simulink model "in_search_for_controller"  (R2017b)
settings: Solver=FixedStepDiscrete  StartTime=0.0  StopTime=10  FixedStep=0.01  RelTol=1e-3
undefined symbols (not defined in the file): g, h, lf, lr, m, r, wf, wr
libraries: vrlib x4, simulink x3, sharedtransform x1
settings Model: Creator=ashwin.ramanujam  LastModifiedBy=Lenovo g505s
settings DataIOCC: ReturnWorkspaceOutputs=on

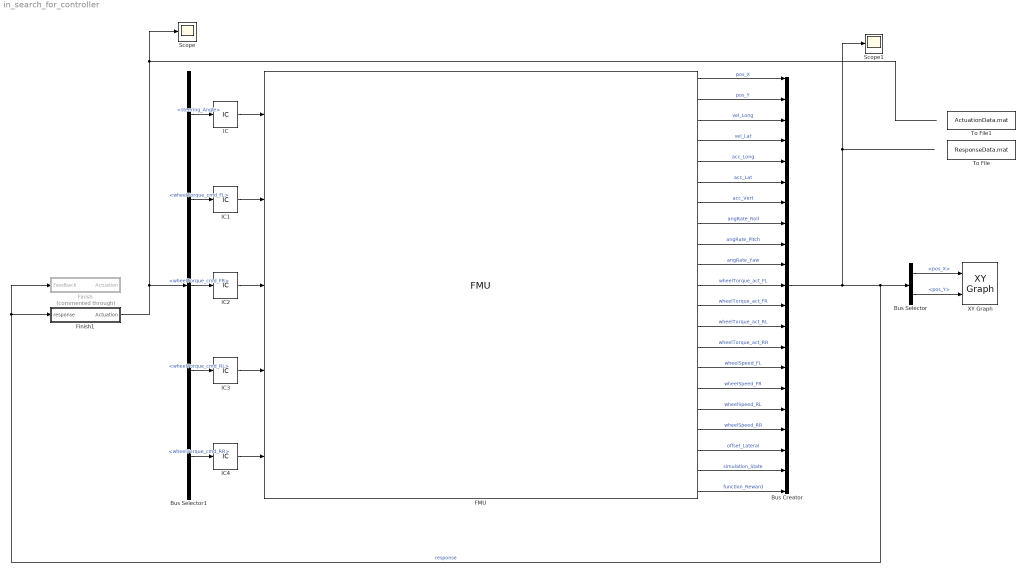
== system in_search_for_controller ==
  Bus Creator : BusCreator  Inputs=21  OutDataTypeStr=Bus: response
  Bus Selector : BusSelector  OutputSignals=pos_X,pos_Y
  Bus Selector1 : BusSelector  OutputSignals=steering_Angle,wheelTorque_cmd_FL,wheelTorque_cmd_FR,wheelTorque_cmd_RL,wheelTorque_cmd_RR
  FMU : FMU  FMUName=MED2018_VehicleModel.fmu  FMUDebugLogging=on  FMUMode=CoSimulation  FMUSampleTime=-1  mask(MED2018.VehicleModel [Co-Simulation, v2.0]){}
      mask Display:
      | if (exist([Simulink.fileGenControl('get','CacheFolder') '\slprj\_fmu\c29ffcaf52b39851ed42bd800156c3ac\MED2018_VehicleModel\model.png'],'file'))
      |     image([Simulink.fileGenControl('get','CacheFolder') '\slprj\_fmu\c29ffcaf52b39851ed42bd800156c3ac\MED2018_VehicleModel\model.png']);
      |     text(0.03, 0.97, 'MED2018.VehicleModel', 'horizontalAlignment', 'left', 'verticalAlignment', 'top');
      | else
      |     disp('MED2018.VehicleModel');
      | end
      | port_label('output',1,'pos_X');
      | port_label('output',2,'pos_Y');
      | port_label('output',3,'vel_Long');
      | port_label('output',4,'vel_Lat');
      | port_label('output',5,'acc_Long');
      | port_label('output',6,'acc_Lat');
      | port_label('output',7,'acc_Vert');
      | port_label('output',8,'angRate_Roll');
      | port_label('output',9,'angRate_Pitch');
      | port_label('output',10,'angRate_Yaw');
      | port_label('output',11,'wheellTorque_act_FL');
      | port_label('output',12,'wheelTorque_act_FR');
      | port_label('output',13,'wheelTorque_act_RL');
      | port_label('output',14,'wheelTorque_act_RR');
      | port_label('output',15,'wheelSpeed_FL');
      | port_label('output',16,'wheelSpeed_FR');
      | port_label('output',17,'wheelSpeed_RL');
      | port_label('output',18,'wheelSpeed_RR');
      | port_label('output',19,'offset_Lateral');
      | port_label('output',20,'simulation_State');
      | port_label('output',21,'function_Reward');
      | port_label('input',1,'steering_Angle');
      | port_label('input',2,'wheelTorque_cmd_FL');
      | port_label('input',3,'wheelTorque_cmd_FR');
      | port_label('input',4,'wheelTorque_cmd_RL');
      | port_label('input',5,'wheelTorque_cmd_RR');
  Finish : Subsystem  Commented=through
  Finish1 : Subsystem
  IC{,1..4} (5 alike) : InitialCondition  Value=0
  Scope : Scope
  Scope1 : Scope
  To File : ToFile  Filename=ResponseData.mat  SaveFormat=Timeseries
  To File1 : ToFile  Filename=ActuationData.mat  SaveFormat=Timeseries
  XY Graph : simulink/Sinks/XY Graph  xmin=-10  xmax=160  ymin=-80  ymax=80  st=-1
  wires:
  Bus Selector1/1 -> IC/1  "<steering_Angle>"
  Bus Selector1/2 -> IC1/1  "<wheelTorque_cmd_FL>"
  Bus Selector1/3 -> IC2/1  "<wheelTorque_cmd_FR>"
  Bus Selector1/4 -> IC3/1  "<wheelTorque_cmd_RL>"
  Bus Selector1/5 -> IC4/1  "<wheelTorque_cmd_RR>"
  FMU/1 -> Bus Creator/1  "pos_X"
  FMU/2 -> Bus Creator/2  "pos_Y"
  FMU/3 -> Bus Creator/3  "vel_Long"
  FMU/4 -> Bus Creator/4  "vel_Lat"
  FMU/5 -> Bus Creator/5  "acc_Long"
  FMU/6 -> Bus Creator/6  "acc_Lat"
  FMU/7 -> Bus Creator/7  "acc_Vert"
  FMU/8 -> Bus Creator/8  "angRate_Roll"
  FMU/9 -> Bus Creator/9  "angRate_Pitch"
  FMU/10 -> Bus Creator/10  "angRate_Yaw"
  FMU/11 -> Bus Creator/11  "wheelTorque_act_FL"
  FMU/12 -> Bus Creator/12  "wheelTorque_act_FR"
  FMU/13 -> Bus Creator/13  "wheelTorque_act_RL"
  FMU/14 -> Bus Creator/14  "wheelTorque_act_RR"
  FMU/15 -> Bus Creator/15  "wheelSpeed_FL"
  FMU/16 -> Bus Creator/16  "wheelSpeed_FR"
  FMU/17 -> Bus Creator/17  "wheelSpeed_RL"
  FMU/18 -> Bus Creator/18  "wheelSpeed_RR"
  FMU/19 -> Bus Creator/19  "offset_Lateral"
  FMU/20 -> Bus Creator/20  "simulation_State"
  FMU/21 -> Bus Creator/21  "function_Reward"
  Bus Selector/1 -> XY Graph/1  "<pos_X>"
  Bus Selector/2 -> XY Graph/2  "<pos_Y>"
  Bus Creator/1 -> Scope1/1, Finish1/1(response), Finish/1(Feedback), Bus Selector/1  "response"
  Finish1/1(Actuation) -> Bus Selector1/1, Scope/1
  IC/1 -> FMU/1
  IC1/1 -> FMU/2
  IC2/1 -> FMU/3
  IC3/1 -> FMU/4
  IC4/1 -> FMU/5

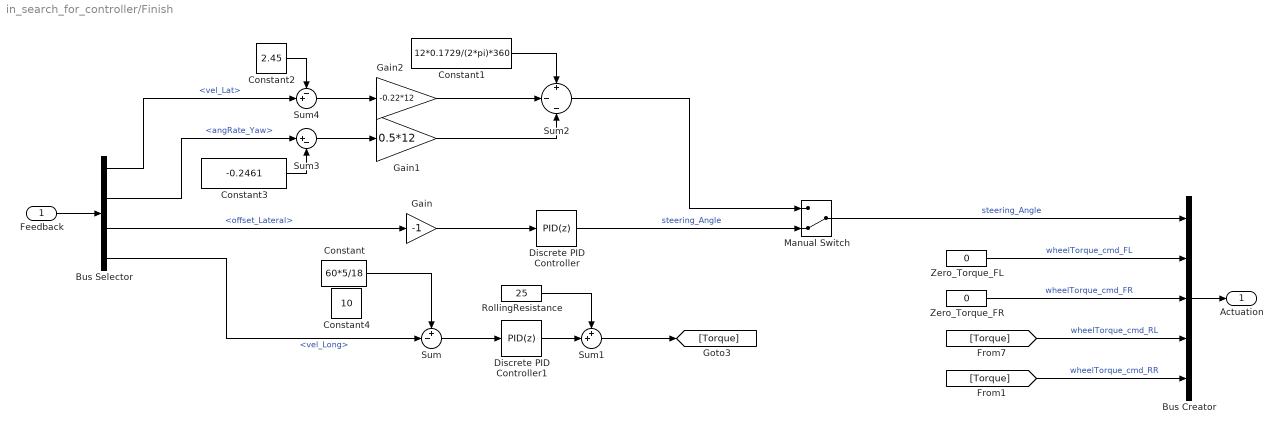
== system in_search_for_controller/Finish ==
  Feedback : Inport
  Bus Creator : BusCreator  Inputs=5
  Bus Selector : BusSelector  OutputSignals=vel_Lat,angRate_Yaw,offset_Lateral,vel_Long
  Constant : Constant  Value=60*5/18
  Constant1 : Constant  Value=12*0.1729/(2*pi)*360
  Constant2 : Constant  Value=2.45
  Constant3 : Constant  Value=-0.2461
  Constant4 : Constant  Value=10
  Discrete PID Controller : simulink/Continuous/PID Controller  Controller=PID  TimeDomain=Discrete-time  SampleTime=-1  IntegratorMethod=Forward Euler  FilterMethod=Forward Euler  Form=Parallel  UseFilter=off  ControllerParametersSource=internal  P=1  I=0  D=1  N=100  InitialConditionSource=internal  InitialConditionForIntegrator=0  InitialConditionForFilter=0  ExternalReset=none  LimitOutput=off  UpperSaturationLimit=inf  LowerSaturationLimit=-inf  LinearizeAsGain=off  AntiWindupMode=none  Kb=1  TrackingMode=off  Kt=1  PParamMin=[]  PParamMax=[]  IParamMin=[]  IParamMax=[]  DParamMin=[]  DParamMax=[]  NParamMin=[]  NParamMax=[]  KbParamMin=[]  KbParamMax=[]  KtParamMin=[]  KtParamMax=[]  POutMin=[]  POutMax=[]  IOutMin=[]  IOutMax=[]  DOutMin=[]  DOutMax=[]  NOutMin=[]  NOutMax=[]  KbOutMin=[]  KbOutMax=[]  KtOutMin=[]  KtOutMax=[]  IntegratorOutMin=[]  IntegratorOutMax=[]  FilterOutMin=[]  FilterOutMax=[]  SumOutMin=[]  SumOutMax=[]  SumI1OutMin=[]  SumI1OutMax=[]  SumI2OutMin=[]  SumI2OutMax=[]  SumI3OutMin=[]  SumI3OutMax=[]  SumDOutMin=[]  SumDOutMax=[]  SaturationOutMin=[]  SaturationOutMax=[]  IntegratorContinuousStateAttributes=''  IntegratorStateMustResolveToSignalObject=off  IntegratorRTWStateStorageClass=Auto  FilterContinuousStateAttributes=''  FilterStateMustResolveToSignalObject=off  FilterRTWStateStorageClass=Auto  DifferentiatorICPrevScaledInput=0  DifferentiatorOutMin=[]  DifferentiatorOutMax=[]  InitialConditionSetting=State (most efficient)  FilterDiffOutCoefMin=[]  FilterDiffOutCoefMax=[]  SumDenOutMin=[]  SumDenOutMax=[]  SumNumOutMin=[]  SumNumOutMax=[]  ReciprocalOutMin=[]  ReciprocalOutMax=[]  DivideOutMin=[]  DivideOutMax=[]  TunerSelectOption=Transfer Function Based (PID Tuner App)
  Discrete PID Controller1 : simulink/Continuous/PID Controller  Controller=PID  TimeDomain=Discrete-time  SampleTime=-1  IntegratorMethod=Forward Euler  FilterMethod=Forward Euler  Form=Parallel  UseFilter=on  ControllerParametersSource=internal  P=100  I=0  D=0.1  N=100  InitialConditionSource=internal  InitialConditionForIntegrator=0  InitialConditionForFilter=0  ExternalReset=none  LimitOutput=off  UpperSaturationLimit=inf  LowerSaturationLimit=-inf  LinearizeAsGain=off  AntiWindupMode=none  Kb=1  TrackingMode=off  Kt=1  PParamMin=[]  PParamMax=[]  IParamMin=[]  IParamMax=[]  DParamMin=[]  DParamMax=[]  NParamMin=[]  NParamMax=[]  KbParamMin=[]  KbParamMax=[]  KtParamMin=[]  KtParamMax=[]  POutMin=[]  POutMax=[]  IOutMin=[]  IOutMax=[]  DOutMin=[]  DOutMax=[]  NOutMin=[]  NOutMax=[]  KbOutMin=[]  KbOutMax=[]  KtOutMin=[]  KtOutMax=[]  IntegratorOutMin=[]  IntegratorOutMax=[]  FilterOutMin=[]  FilterOutMax=[]  SumOutMin=[]  SumOutMax=[]  SumI1OutMin=[]  SumI1OutMax=[]  SumI2OutMin=[]  SumI2OutMax=[]  SumI3OutMin=[]  SumI3OutMax=[]  SumDOutMin=[]  SumDOutMax=[]  SaturationOutMin=[]  SaturationOutMax=[]  IntegratorContinuousStateAttributes=''  IntegratorStateMustResolveToSignalObject=off  IntegratorRTWStateStorageClass=Auto  FilterContinuousStateAttributes=''  FilterStateMustResolveToSignalObject=off  FilterRTWStateStorageClass=Auto  DifferentiatorICPrevScaledInput=0  DifferentiatorOutMin=[]  DifferentiatorOutMax=[]  InitialConditionSetting=State (most efficient)  FilterDiffOutCoefMin=[]  FilterDiffOutCoefMax=[]  SumDenOutMin=[]  SumDenOutMax=[]  SumNumOutMin=[]  SumNumOutMax=[]  ReciprocalOutMin=[]  ReciprocalOutMax=[]  DivideOutMin=[]  DivideOutMax=[]  TunerSelectOption=Transfer Function Based (PID Tuner App)
  Gain : Gain  Gain=-1
  Gain1 : Gain  Gain=0.5*12
  Gain2 : Gain  Gain=-0.22*12
  Manual Switch : ManualSwitch  CurrentSetting=0
  RollingResistance : Constant  Value=25
  Sum : Sum  Inputs=+-|
  Sum1 : Sum  Inputs=++|
  Sum2 : Sum  Inputs=+|-|-
  Sum3 : Sum  Inputs=|+-
  Sum4 : Sum  Inputs=-+|
  Zero_Torque_FL : Constant  Value=0
  Zero_Torque_FR : Constant  Value=0
  Actuation : Outport
  wires:
  Bus Creator/1 -> Actuation/1
  Gain/1 -> Discrete PID Controller/1
  Sum/1 -> Discrete PID Controller1/1
  Feedback/1 -> Bus Selector/1
  Sum1/1 -> [Torque]
  Bus Selector/4 -> Sum/2  "<vel_Long>"
  Bus Selector/3 -> Gain/1  "<offset_Lateral>"
  Manual Switch/1 -> Bus Creator/1  "steering_Angle"
  Discrete PID Controller1/1 -> Sum1/2
  RollingResistance/1 -> Sum1/1
  Zero_Torque_FL/1 -> Bus Creator/2  "wheelTorque_cmd_FL"
  [Torque] -> Bus Creator/4  "wheelTorque_cmd_RL"
  Zero_Torque_FR/1 -> Bus Creator/3  "wheelTorque_cmd_FR"
  [Torque] -> Bus Creator/5  "wheelTorque_cmd_RR"
  Gain1/1 -> Sum2/3
  Gain2/1 -> Sum2/2
  Constant1/1 -> Sum2/1
  Sum4/1 -> Gain2/1
  Sum3/1 -> Gain1/1
  Constant2/1 -> Sum4/1
  Constant3/1 -> Sum3/2
  Bus Selector/2 -> Sum3/1  "<angRate_Yaw>"
  Bus Selector/1 -> Sum4/2  "<vel_Lat>"
  Discrete PID Controller/1 -> Manual Switch/2  "steering_Angle"
  Constant/1 -> Sum/1
  Sum2/1 -> Manual Switch/1

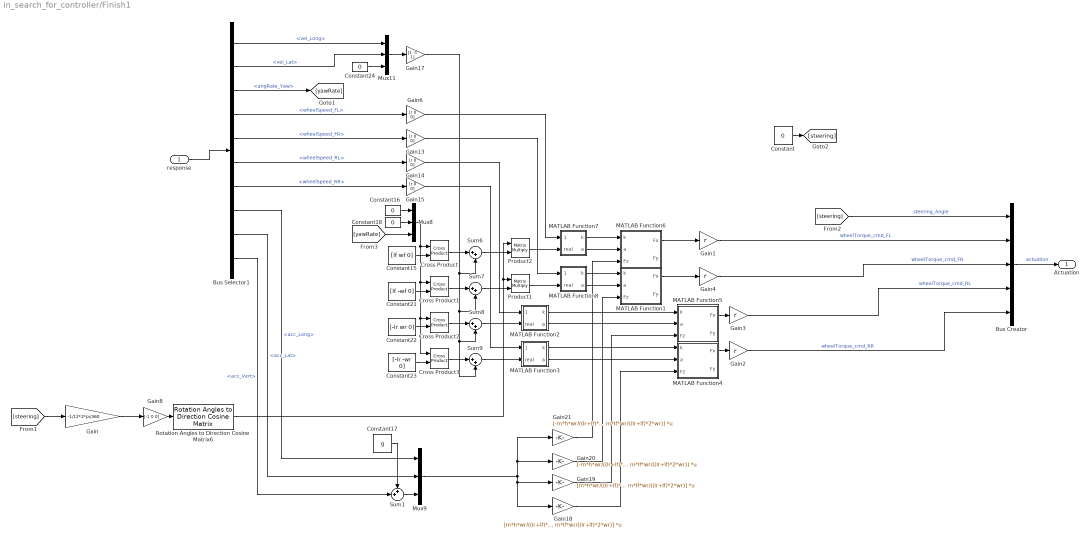
== system in_search_for_controller/Finish1 ==
  response : Inport
  Bus Creator : BusCreator  Inputs=5  OutDataTypeStr=Bus: actuation
  Bus Selector1 : BusSelector  OutputSignals=vel_Long,vel_Lat,angRate_Yaw,wheelSpeed_FL,wheelSpeed_FR,wheelSpeed_RL,wheelSpeed_RR,acc_Long,acc_Lat,acc_Vert
  Constant{,16,18,24} (4 alike) : Constant  Value=0
  Constant15 : Constant  Value=[lf wf 0]
  Constant17 : Constant  Value=g
  Constant21 : Constant  Value=[lf -wf 0]
  Constant22 : Constant  Value=[-lr wr 0]
  Constant23 : Constant  Value=[-lr -wr 0]
  Cross Product{,1..3} (4 alike) : vrlib/Utilities/Cross Product
      settings: SourceProductBaseCode=VR
  Gain : Gain  Gain=-1/12*2*pi/360
  Gain{1..4} (4 alike) : Gain  Gain=r
  Gain{6,13..15} (4 alike) : Gain  Gain=[r 0 0]
  Gain17 : Gain  Gain=[1 -1 1]
  Gain18 : Gain  Gain=[m*h*wr/((lr+lf)*2*wr) m*h*lf/((lr+lf)*2*wr) m*lf*wr/((lr+lf)*2*wr)]  Multiplication=Matrix(K*u)
  Gain19 : Gain  Gain=[m*h*wr/((lr+lf)*2*wr) -m*h*lf/((lr+lf)*2*wr) m*lf*wr/((lr+lf)*2*wr)]  Multiplication=Matrix(K*u)
  Gain20 : Gain  Gain=[-m*h*wr/((lr+lf)*2*wr) m*h*lf/((lr+lf)*2*wr) m*lf*wr/((lr+lf)*2*wr)]  Multiplication=Matrix(K*u)
  Gain21 : Gain  Gain=[-m*h*wr/((lr+lf)*2*wr) -m*h*lf/((lr+lf)*2*wr) m*lf*wr/((lr+lf)*2*wr)]  Multiplication=Matrix(K*u)
  Gain8 : Gain  Gain=[-1 0 0]
  MATLAB Function1 : MATLAB Function  TreatAsAtomicUnit=on
  MATLAB Function2 : MATLAB Function  TreatAsAtomicUnit=on
  MATLAB Function3 : MATLAB Function  TreatAsAtomicUnit=on
  MATLAB Function4 : MATLAB Function  TreatAsAtomicUnit=on
  MATLAB Function5 : MATLAB Function  TreatAsAtomicUnit=on
  MATLAB Function6 : MATLAB Function  TreatAsAtomicUnit=on
  MATLAB Function7 : MATLAB Function  TreatAsAtomicUnit=on
  MATLAB Function8 : MATLAB Function  TreatAsAtomicUnit=on
  Mux11 : Mux  Inputs=3
  Mux8 : Mux  Inputs=3
  Mux9 : Mux  Inputs=3
  Product1 : Product  Multiplication=Matrix(*)
  Product2 : Product  Multiplication=Matrix(*)
  Rotation Angles to Direction Cosine Matrix6 : sharedtransform/Rotation Angles to Direction Cosine Matrix  rotationOrder=ZYX
      settings: SourceProductBaseCode=AE
  Sum1 : Sum  Inputs=++|
  Sum{6..9} (4 alike) : Sum  Inputs=|++
  Actuation : Outport
  wires:
  Bus Creator/1 -> Actuation/1  "actuation"
  [steering] -> Bus Creator/1  "steering_Angle"
  Gain1/1 -> Bus Creator/2  "wheelTorque_cmd_FL"
  Gain3/1 -> Bus Creator/4  "wheelTorque_cmd_RL"
  Gain4/1 -> Bus Creator/3  "wheelTorque_cmd_FR"
  Gain2/1 -> Bus Creator/5  "wheelTorque_cmd_RR"
  Mux11/1 -> Gain17/1
  Constant15/1 -> Cross Product/2
  Gain13/1 -> MATLAB Function8/1(requ)
  Sum9/1 -> MATLAB Function3/2(real)
  MATLAB Function8/1(k) -> MATLAB Function1/1(k)
  Product2/1 -> MATLAB Function7/2(real)
  Gain14/1 -> MATLAB Function2/1(requ)
  Cross Product2/1 -> Sum8/1
  Gain6/1 -> MATLAB Function7/1(requ)
  Bus Selector1/8 -> Mux9/1  "<acc_Long>"
  Sum6/1 -> Product2/2
  Sum8/1 -> MATLAB Function2/2(real)
  Sum7/1 -> Product1/2
  Gain18/1 -> MATLAB Function4/3(Fz)
  Cross Product/1 -> Sum6/1
  MATLAB Function2/2(a) -> MATLAB Function5/2(a)
  MATLAB Function3/1(k) -> MATLAB Function4/1(k)
  MATLAB Function3/2(a) -> MATLAB Function4/2(a)
  Gain17/1 -> Sum9/2, Sum8/2, Sum7/2, Sum6/2
  Gain19/1 -> MATLAB Function5/3(Fz)
  Rotation Angles to Direction Cosine Matrix6/1 -> Product2/1, Product1/1
  MATLAB Function2/1(k) -> MATLAB Function5/1(k)
  Gain/1 -> Gain8/1
  Constant21/1 -> Cross Product1/2
  Constant23/1 -> Cross Product3/2
  MATLAB Function7/2(a) -> MATLAB Function6/2(a)
  Gain8/1 -> Rotation Angles to Direction Cosine Matrix6/1
  [yawRate] -> Mux8/3
  Gain15/1 -> MATLAB Function3/1(requ)
  Bus Selector1/7 -> Gain15/1  "<wheelSpeed_RR>"
  Gain20/1 -> MATLAB Function1/3(Fz)
  Product1/1 -> MATLAB Function8/2(real)
  Bus Selector1/10 -> Sum1/2  "<acc_Vert>"
  Cross Product1/1 -> Sum7/1
  Mux8/1 -> Cross Product/1, Cross Product2/1, Cross Product3/1, Cross Product1/1
  MATLAB Function8/2(a) -> MATLAB Function1/2(a)
  Cross Product3/1 -> Sum9/1
  Constant16/1 -> Mux8/1
  MATLAB Function7/1(k) -> MATLAB Function6/1(k)
  Bus Selector1/4 -> Gain6/1  "<wheelSpeed_FL>"
  Constant22/1 -> Cross Product2/2
  Mux9/1 -> Gain18/1, Gain19/1, Gain21/1, Gain20/1
  Bus Selector1/6 -> Gain14/1  "<wheelSpeed_RL>"
  Constant17/1 -> Sum1/1
  Constant24/1 -> Mux11/3
  Constant18/1 -> Mux8/2
  Bus Selector1/3 -> [yawRate]  "<angRate_Yaw>"
  Sum1/1 -> Mux9/3
  Bus Selector1/2 -> Mux11/2  "<vel_Lat>"
  response/1 -> Bus Selector1/1
  Gain21/1 -> MATLAB Function6/3(Fz)
  Bus Selector1/9 -> Mux9/2  "<acc_Lat>"
  Bus Selector1/1 -> Mux11/1  "<vel_Long>"
  Bus Selector1/5 -> Gain13/1  "<wheelSpeed_FR>"
  [steering] -> Gain/1
  Constant/1 -> [steering]
  MATLAB Function6/1(Fx) -> Gain1/1
  MATLAB Function5/1(Fx) -> Gain3/1
  MATLAB Function4/1(Fx) -> Gain2/1
  MATLAB Function1/1(Fx) -> Gain4/1

== matlab function in_search_for_controller/Finish1/MATLAB Function1 ==
  data: k input; Fx output; a input; Fz input; Fy output
function [Fx, Fy] = F_x(k, a, Fz)
a=-a;
Fz0 = 3124;
PCX1=1.63;
PDX1=1.06;
PDX2=-0.0492;
PEX1=0.5;
PEX2=-0.11;
PEX3=-0.06;
PEX4=0;
PKX1=19.7;
PKX2=-0.15;
PKX3=0.18;
PHX1=-0.0005;
PHX2=8.5e-5;
PVX1=0;
PVX2=0;
RBX1=9.0;
RBX2=-8.6;
RCX1=1.131;
REX1=0.081;
REX2=-0.15;
RHX1=-0.029;
PCY1=1.28;
PDY1=-0.92;
PDY2=0.22;
PEY1=-1.1;
PEY2=0.65;
PEY3=-0.65;
PKY1=-13.06;
PKY2=1.77;
PHY1=0.0034;
PHY2=-0.003;
PVY1=0.044;
PVY2=-0.030;
RBY1=6.4;
RBY2=7.91;
RBY3=-0.059;
RCY1=1.16;
REY1=0.22;
REY2=0.43;
RHY1=0.0007;
RHY2=0.023;
RVY1=0;
RVY2=0;
RVY4=10;
RVY5=1.94;
RVY6=-50;
 
%k = w*Re/Vx - 1;
dfz = (Fz - Fz0)/Fz0;

Shx = PHX1 + PHX2*dfz;
Svx = Fz * (PVX1 + PVX2 * dfz);
kx = k + Shx;
Cx = PCX1;
Dx = Fz*(PDX1 + PDX2 * dfz);
Ex = (PEX1 + PEX2 * dfz + PEX3 * dfz^2) * (1 - PEX4 * sign(kx));
Bx = Fz * (PKX1 + PKX2 * dfz) * exp(PKX3 * dfz) / (Cx*Dx);
Fx0 = Dx*sin(Cx*atan(Bx*kx - Ex*(Bx*kx - atan(Bx*kx)))) + Svx;

Bxa = RBX1 * cos(atan(RBX2 * k));
Cxa = RCX1;
Exa = REX1 + REX2*dfz;
Shxa = RHX1;
as = a + Shxa;
Gxa = (cos(Cxa*atan(Bxa*as - Exa*(Bxa*as - atan(Bxa*as)))))/...
(cos(Cxa*atan(Bxa*Shxa - Exa*(Bxa*Shxa - atan(Bxa*Shxa)))));

Fx = Fx0 * Gxa;


Shy = PHY1 + PHY2*dfz;
Svy = Fz * (PVY1 + PVY2 * dfz);
ay = a + Shy;
Cy = PCY1;
Dy = Fz*(PDY1 + PDY2 * dfz);
Ey = (PEY1 + PEY2 * dfz) * (1 - PEY3 * sign(ay));
By = PKY1 * Fz0 * sin(2 * atan(Fz/(PKY2 * Fz0)))  / (Cy*Dy);
Fy0 = Dy*sin(Cy*atan(By*ay - Ey*(By*ay - atan(By*ay)))) + Svy;

Svyk = (PDY1 + PDY2*dfz) *Fz*(RVY1 + RVY2*dfz)*...
    cos(atan(RVY4*a))*sin(RVY5 * atan(RVY6*k));
Shyk = RHY1 + RHY2 * dfz;
ks = k + Shyk;
Byk = RBY1 * cos(atan(RBY2 * (a - RBY3)));
Cyk = RCY1;
Eyk = REY1 + REY2*dfz;
Gyk = (cos(Cyk*atan(Byk*ks - Eyk*(Byk*ks - atan(Byk*ks)))))/...
(cos(Cyk*atan(Byk*Shyk - Eyk*(Byk*Shyk - atan(Byk*Shyk)))));

Fy = -(Fy0 * Gyk + Svyk);
end

== matlab function in_search_for_controller/Finish1/MATLAB Function6 ==
  data: k input; Fx output; a input; Fz input; Fy output
function [Fx, Fy] = F_x(k, a, Fz)
Fz0 = 3124;
PCX1=1.63;
PDX1=1.06;
PDX2=-0.0492;
PEX1=0.5;
PEX2=-0.11;
PEX3=-0.06;
PEX4=0;
PKX1=19.7;
PKX2=-0.15;
PKX3=0.18;
PHX1=-0.0005;
PHX2=8.5e-5;
PVX1=0;
PVX2=0;
RBX1=9.0;
RBX2=-8.6;
RCX1=1.131;
REX1=0.081;
REX2=-0.15;
RHX1=-0.029;
PCY1=1.28;
PDY1=-0.92;
PDY2=0.22;
PEY1=-1.1;
PEY2=0.65;
PEY3=-0.65;
PKY1=-13.06;
PKY2=1.77;
PHY1=0.0034;
PHY2=-0.003;
PVY1=0.044;
PVY2=-0.030;
RBY1=6.4;
RBY2=7.91;
RBY3=-0.059;
RCY1=1.16;
REY1=0.22;
REY2=0.43;
RHY1=0.0007;
RHY2=0.023;
RVY1=0;
RVY2=0;
RVY4=10;
RVY5=1.94;
RVY6=-50;
 
%k = w*Re/Vx - 1;
dfz = (Fz - Fz0)/Fz0;

Shx = PHX1 + PHX2*dfz;
Svx = Fz * (PVX1 + PVX2 * dfz);
kx = k + Shx;
Cx = PCX1;
Dx = Fz*(PDX1 + PDX2 * dfz);
Ex = (PEX1 + PEX2 * dfz + PEX3 * dfz^2) * (1 - PEX4 * sign(kx));
Bx = Fz * (PKX1 + PKX2 * dfz) * exp(PKX3 * dfz) / (Cx*Dx);
Fx0 = Dx*sin(Cx*atan(Bx*kx - Ex*(Bx*kx - atan(Bx*kx)))) + Svx;

Bxa = RBX1 * cos(atan(RBX2 * k));
Cxa = RCX1;
Exa = REX1 + REX2*dfz;
Shxa = RHX1;
as = a + Shxa;
Gxa = (cos(Cxa*atan(Bxa*as - Exa*(Bxa*as - atan(Bxa*as)))))/...
(cos(Cxa*atan(Bxa*Shxa - Exa*(Bxa*Shxa - atan(Bxa*Shxa)))));

Fx = Fx0 * Gxa;


Shy = PHY1 + PHY2*dfz;
Svy = Fz * (PVY1 + PVY2 * dfz);
ay = a + Shy;
Cy = PCY1;
Dy = Fz*(PDY1 + PDY2 * dfz);
Ey = (PEY1 + PEY2 * dfz) * (1 - PEY3 * sign(ay));
By = PKY1 * Fz0 * sin(2 * atan(Fz/(PKY2 * Fz0)))  / (Cy*Dy);
Fy0 = Dy*sin(Cy*atan(By*ay - Ey*(By*ay - atan(By*ay)))) + Svy;

Svyk = (PDY1 + PDY2*dfz) *Fz*(RVY1 + RVY2*dfz)*...
    cos(atan(RVY4*a))*sin(RVY5 * atan(RVY6*k));
Shyk = RHY1 + RHY2 * dfz;
ks = k + Shyk;
Byk = RBY1 * cos(atan(RBY2 * (a - RBY3)));
Cyk = RCY1;
Eyk = REY1 + REY2*dfz;
Gyk = (cos(Cyk*atan(Byk*ks - Eyk*(Byk*ks - atan(Byk*ks)))))/...
(cos(Cyk*atan(Byk*Shyk - Eyk*(Byk*Shyk - atan(Byk*Shyk)))));

Fy = Fy0 * Gyk + Svyk;
end

== matlab function in_search_for_controller/Finish1/MATLAB Function2 ==
  data: requ input; k output; real input; a output
function [k, a] = fcn(requ, real)
a = atan2(real(2), real(1));
k = (requ(1) - real(1))/real(1);
end

== matlab function in_search_for_controller/Finish1/MATLAB Function3 ==
  data: requ input; k output; real input; a output
function [k, a] = fcn(requ, real)
a = atan2(real(2), real(1));
k = (requ(1) - real(1))/real(1);
end

== matlab function in_search_for_controller/Finish1/MATLAB Function4 ==
  data: k input; Fx output; a input; Fz input; Fy output
function [Fx, Fy] = F_x(k, a, Fz)
a=-a;
Fz0 = 3252;
PCX1=1.63;
PDX1=1.06;
PDX2=-0.0492;
PEX1=0.5;
PEX2=-0.11;
PEX3=-0.06;
PEX4=0;
PKX1=19.7;
PKX2=-0.15;
PKX3=0.18;
PHX1=-0.0005;
PHX2=8.5e-5;
PVX1=0;
PVX2=0;
RBX1=9.0;
RBX2=-8.6;
RCX1=1.131;
REX1=0.081;
REX2=-0.15;
RHX1=-0.029;
PCY1=1.28;
PDY1=-0.92;
PDY2=0.22;
PEY1=-1.1;
PEY2=0.65;
PEY3=-0.65;
PKY1=-13.06;
PKY2=1.77;
PHY1=0.0034;
PHY2=-0.003;
PVY1=0.044;
PVY2=-0.030;
RBY1=6.4;
RBY2=7.91;
RBY3=-0.059;
RCY1=1.16;
REY1=0.22;
REY2=0.43;
RHY1=0.0007;
RHY2=0.023;
RVY1=0;
RVY2=0;
RVY4=10;
RVY5=1.94;
RVY6=-50;
 
%k = w*Re/Vx - 1;
dfz = (Fz - Fz0)/Fz0;

Shx = PHX1 + PHX2*dfz;
Svx = Fz * (PVX1 + PVX2 * dfz);
kx = k + Shx;
Cx = PCX1;
Dx = Fz*(PDX1 + PDX2 * dfz);
Ex = (PEX1 + PEX2 * dfz + PEX3 * dfz^2) * (1 - PEX4 * sign(kx));
Bx = Fz * (PKX1 + PKX2 * dfz) * exp(PKX3 * dfz) / (Cx*Dx);
Fx0 = Dx*sin(Cx*atan(Bx*kx - Ex*(Bx*kx - atan(Bx*kx)))) + Svx;

Bxa = RBX1 * cos(atan(RBX2 * k));
Cxa = RCX1;
Exa = REX1 + REX2*dfz;
Shxa = RHX1;
as = a + Shxa;
Gxa = (cos(Cxa*atan(Bxa*as - Exa*(Bxa*as - atan(Bxa*as)))))/...
(cos(Cxa*atan(Bxa*Shxa - Exa*(Bxa*Shxa - atan(Bxa*Shxa)))));

Fx = Fx0 * Gxa;


Shy = PHY1 + PHY2*dfz;
Svy = Fz * (PVY1 + PVY2 * dfz);
ay = a + Shy;
Cy = PCY1;
Dy = Fz*(PDY1 + PDY2 * dfz);
Ey = (PEY1 + PEY2 * dfz) * (1 - PEY3 * sign(ay));
By = PKY1 * Fz0 * sin(2 * atan(Fz/(PKY2 * Fz0)))  / (Cy*Dy);
Fy0 = Dy*sin(Cy*atan(By*ay - Ey*(By*ay - atan(By*ay)))) + Svy;

Svyk = (PDY1 + PDY2*dfz) *Fz*(RVY1 + RVY2*dfz)*...
    cos(atan(RVY4*a))*sin(RVY5 * atan(RVY6*k));
Shyk = RHY1 + RHY2 * dfz;
ks = k + Shyk;
Byk = RBY1 * cos(atan(RBY2 * (a - RBY3)));
Cyk = RCY1;
Eyk = REY1 + REY2*dfz;
Gyk = (cos(Cyk*atan(Byk*ks - Eyk*(Byk*ks - atan(Byk*ks)))))/...
(cos(Cyk*atan(Byk*Shyk - Eyk*(Byk*Shyk - atan(Byk*Shyk)))));

Fy = -(Fy0 * Gyk + Svyk);
end

== matlab function in_search_for_controller/Finish1/MATLAB Function5 ==
  data: k input; Fx output; a input; Fz input; Fy output
function [Fx, Fy] = F_x(k, a, Fz)
Fz0 = 3252;
PCX1=1.63;
PDX1=1.06;
PDX2=-0.0492;
PEX1=0.5;
PEX2=-0.11;
PEX3=-0.06;
PEX4=0;
PKX1=19.7;
PKX2=-0.15;
PKX3=0.18;
PHX1=-0.0005;
PHX2=8.5e-5;
PVX1=0;
PVX2=0;
RBX1=9.0;
RBX2=-8.6;
RCX1=1.131;
REX1=0.081;
REX2=-0.15;
RHX1=-0.029;
PCY1=1.28;
PDY1=-0.92;
PDY2=0.22;
PEY1=-1.1;
PEY2=0.65;
PEY3=-0.65;
PKY1=-13.06;
PKY2=1.77;
PHY1=0.0034;
PHY2=-0.003;
PVY1=0.044;
PVY2=-0.030;
RBY1=6.4;
RBY2=7.91;
RBY3=-0.059;
RCY1=1.16;
REY1=0.22;
REY2=0.43;
RHY1=0.0007;
RHY2=0.023;
RVY1=0;
RVY2=0;
RVY4=10;
RVY5=1.94;
RVY6=-50;
 
%k = w*Re/Vx - 1;
dfz = (Fz - Fz0)/Fz0;

Shx = PHX1 + PHX2*dfz;
Svx = Fz * (PVX1 + PVX2 * dfz);
kx = k + Shx;
Cx = PCX1;
Dx = Fz*(PDX1 + PDX2 * dfz);
Ex = (PEX1 + PEX2 * dfz + PEX3 * dfz^2) * (1 - PEX4 * sign(kx));
Bx = Fz * (PKX1 + PKX2 * dfz) * exp(PKX3 * dfz) / (Cx*Dx);
Fx0 = Dx*sin(Cx*atan(Bx*kx - Ex*(Bx*kx - atan(Bx*kx)))) + Svx;

Bxa = RBX1 * cos(atan(RBX2 * k));
Cxa = RCX1;
Exa = REX1 + REX2*dfz;
Shxa = RHX1;
as = a + Shxa;
Gxa = (cos(Cxa*atan(Bxa*as - Exa*(Bxa*as - atan(Bxa*as)))))/...
(cos(Cxa*atan(Bxa*Shxa - Exa*(Bxa*Shxa - atan(Bxa*Shxa)))));

Fx = Fx0 * Gxa;


Shy = PHY1 + PHY2*dfz;
Svy = Fz * (PVY1 + PVY2 * dfz);
ay = a + Shy;
Cy = PCY1;
Dy = Fz*(PDY1 + PDY2 * dfz);
Ey = (PEY1 + PEY2 * dfz) * (1 - PEY3 * sign(ay));
By = PKY1 * Fz0 * sin(2 * atan(Fz/(PKY2 * Fz0)))  / (Cy*Dy);
Fy0 = Dy*sin(Cy*atan(By*ay - Ey*(By*ay - atan(By*ay)))) + Svy;

Svyk = (PDY1 + PDY2*dfz) *Fz*(RVY1 + RVY2*dfz)*...
    cos(atan(RVY4*a))*sin(RVY5 * atan(RVY6*k));
Shyk = RHY1 + RHY2 * dfz;
ks = k + Shyk;
Byk = RBY1 * cos(atan(RBY2 * (a - RBY3)));
Cyk = RCY1;
Eyk = REY1 + REY2*dfz;
Gyk = (cos(Cyk*atan(Byk*ks - Eyk*(Byk*ks - atan(Byk*ks)))))/...
(cos(Cyk*atan(Byk*Shyk - Eyk*(Byk*Shyk - atan(Byk*Shyk)))));

Fy = Fy0 * Gyk + Svyk;
end

== matlab function in_search_for_controller/Finish1/MATLAB Function7 ==
  data: requ input; k output; real input; a output
function [k, a] = fcn(requ, real)
a = atan2(real(2), real(1));
k = (requ(1) - real(1))/real(1);
end

== matlab function in_search_for_controller/Finish1/MATLAB Function8 ==
  data: requ input; k output; real input; a output
function [k, a] = fcn(requ, real)
a = atan2(real(2), real(1));
k = (requ(1) - real(1))/real(1);
end
